simulink model "example7_1"  (Simulink 8.5)
settings: Solver=ode4  StartTime=0.0  StopTime=10  FixedStep=0.02  RelTol=1e-3
values from neighbouring files (symbols this model uses):
  r = 0.002    [example7_1_fundef.m]    (also in example7_1_solution.m)
settings Model: Creator=chuan  LastModifiedBy=chuan
settings DataIOCC: LimitDataPoints=off  SignalLoggingName=sigsOut
settings OptimizationCC: ExpressionDepthLimit=128
settings DebuggingCC: SaveWithParameterizedLinksMsg=none  SignalResolutionControl=TryResolveAllWithWarning  MultiTaskDSMMsg=warning  MultiTaskCondExecSysMsg=none  FcnCallInpInsideContextMsg=EnableAllAsError  StateNameClashWarn=none  StrictBusMsg=None
settings HardwareCC: TargetUnknown=on

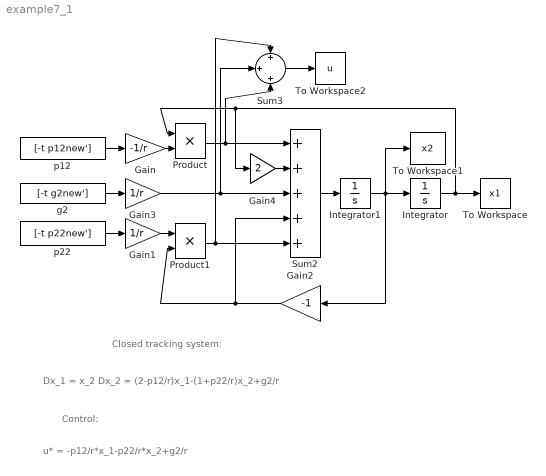
== system example7_1 ==
  note: Closed tracking system:
  note: Dx_1 = x_2
      | Dx_2 = (2-p12/r)x_1-(1+p22/r)x_2+g2/r
  note: Control:
  note: u* = -p12/r*x_1-p22/r*x_2+g2/r
  Gain : Gain  Gain=-1/r  SaturateOnIntegerOverflow=on  OutDataTypeStr=Inherit: Same as input  ParamDataTypeStr=Inherit: Same as input
  Gain1 : Gain  Gain=1/r  SaturateOnIntegerOverflow=on  OutDataTypeStr=Inherit: Same as input  ParamDataTypeStr=Inherit: Same as input
  Gain2 : Gain  Gain=-1  SaturateOnIntegerOverflow=on  OutDataTypeStr=Inherit: Same as input  ParamDataTypeStr=Inherit: Same as input
  Gain3 : Gain  Gain=1/r  SaturateOnIntegerOverflow=on  OutDataTypeStr=Inherit: Same as input  ParamDataTypeStr=Inherit: Same as input
  Gain4 : Gain  Gain=2  SaturateOnIntegerOverflow=on  OutDataTypeStr=Inherit: Same as input  ParamDataTypeStr=Inherit: Same as input
  Integrator : Integrator  InitialCondition=1
  Integrator1 : Integrator  InitialCondition=1
  Product : Product  SaturateOnIntegerOverflow=on  OutDataTypeStr=Inherit: Same as first input
  Product1 : Product  SaturateOnIntegerOverflow=on  OutDataTypeStr=Inherit: Same as first input
  Sum2 : Sum  Inputs=+++++  SaturateOnIntegerOverflow=on
  Sum3 : Sum  Inputs=+|+|+  SaturateOnIntegerOverflow=on
  To Workspace : ToWorkspace  VariableName=x1  SampleTime=-1
  To Workspace1 : ToWorkspace  VariableName=x2  SampleTime=-1
  To Workspace2 : ToWorkspace  VariableName=u  SampleTime=-1
  g2 : FromWorkspace  VariableName=[-t g2new']  SampleTime=0
  p12 : FromWorkspace  VariableName=[-t p12new']  SampleTime=0
  p22 : FromWorkspace  VariableName=[-t p22new']  SampleTime=0
  wires:
  Integrator1/1 -> Gain2/1, Integrator/1, To Workspace1/1
  p12/1 -> Gain/1
  p22/1 -> Gain1/1
  Gain1/1 -> Product1/1
  Gain2/1 -> Product1/2, Sum2/4
  Sum2/1 -> Integrator1/1
  Product/1 -> Sum2/1, Sum3/3
  g2/1 -> Gain3/1
  Gain/1 -> Product/2
  Integrator/1 -> To Workspace/1, Product/1, Gain4/1
  Product1/1 -> Sum2/5, Sum3/1
  Gain3/1 -> Sum2/3, Sum3/2
  Gain4/1 -> Sum2/2
  Sum3/1 -> To Workspace2/1
